simulink model "e05"  (R2023b)
settings: Solver=VariableStepAuto  StartTime=0.0  StopTime=2  RelTol=1e-3
values from neighbouring files (symbols this model uses):
  A = [ ... (first row only)    [e00.m]
  Ad = s1.A    [e00.m]
  B = [ ... (first row only)    [e00.m]
  Bd = s1.B    [e00.m]
  C = [ ... (first row only)    [e00.m]
  Cd = s1.C    [e00.m]
  D = [ ... (first row only)    [e00.m]
  Dd = s1.D    [e00.m]
  Ld = (place(Ad',Cd',p))'    [e00.m]
  Ts = 0.5    [e00.m]
settings Model: Creator=jitbi  LastModifiedBy=Anirvan Krishna

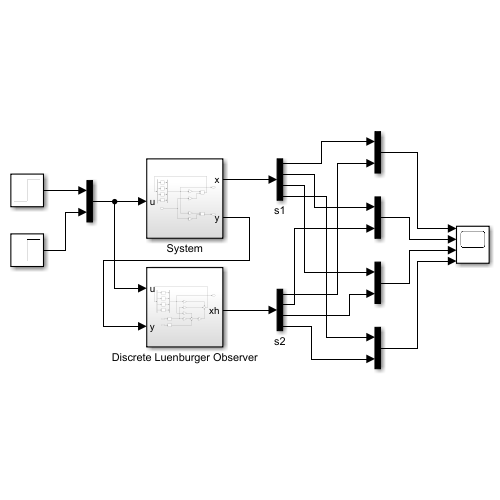
[thumbnail: Simulink's stored preview of the top-level diagram]
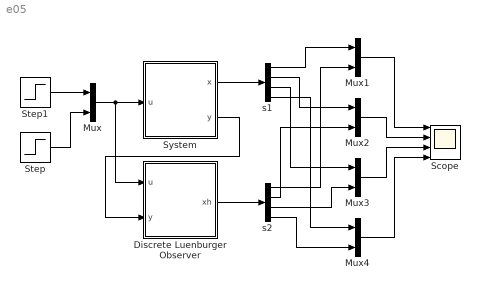
== system e05 ==
  Discrete Luenburger Observer : Subsystem
  Mux{,1..4} (5 alike) : Mux  Inputs=2
  Scope : Scope  NumInputPorts=4
  Step : Step  Time=0  SampleTime=1e-4
  Step1 : Step  Time=0  SampleTime=1e-4
  System : Subsystem
  s1 : Demux
  s2 : Demux
  wires:
  Step/1 -> Mux/2
  Mux/1 -> Discrete Luenburger Observer/1(u), System/1(u)
  Step1/1 -> Mux/1
  System/2(y) -> Discrete Luenburger Observer/2(y)
  System/1(x) -> s1/1
  Discrete Luenburger Observer/1(xh) -> s2/1
  s1/1 -> Mux1/1
  s2/1 -> Mux1/2
  s1/2 -> Mux2/1
  s1/3 -> Mux3/1
  s2/2 -> Mux2/2
  s2/3 -> Mux3/2
  s2/4 -> Mux4/2
  Mux1/1 -> Scope/1
  Mux2/1 -> Scope/2
  Mux3/1 -> Scope/3
  Mux4/1 -> Scope/4
  s1/4 -> Mux4/1

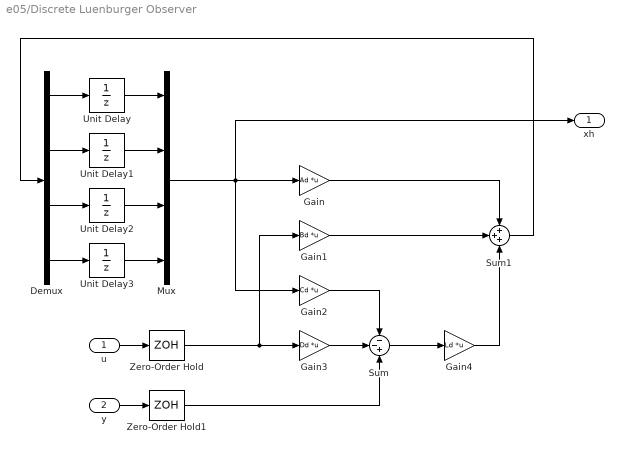
== system e05/Discrete Luenburger Observer ==
  u : Inport
  y : Inport  Port=2
  Demux : Demux
  Gain : Gain  Gain=Ad  Multiplication=Matrix(K*u)
  Gain1 : Gain  Gain=Bd  Multiplication=Matrix(K*u)
  Gain2 : Gain  Gain=Cd  Multiplication=Matrix(K*u)
  Gain3 : Gain  Gain=Dd  Multiplication=Matrix(K*u)
  Gain4 : Gain  Gain=Ld  Multiplication=Matrix(K*u)
  Mux : Mux
  Sum : Sum  Inputs=--+
  Sum1 : Sum  Inputs=+++
  Unit Delay{,1..3} (4 alike) : UnitDelay  SampleTime=Ts  HasFrameUpgradeWarning=on
  Zero-Order Hold : ZeroOrderHold  SampleTime=Ts
  Zero-Order Hold1 : ZeroOrderHold  SampleTime=Ts
  xh : Outport
  wires:
  y/1 -> Zero-Order Hold1/1
  Gain3/1 -> Sum/2
  Unit Delay3/1 -> Mux/4
  Unit Delay1/1 -> Mux/2
  Unit Delay/1 -> Mux/1
  Unit Delay2/1 -> Mux/3
  u/1 -> Zero-Order Hold/1
  Gain4/1 -> Sum1/3
  Demux/2 -> Unit Delay1/1
  Zero-Order Hold/1 -> Gain3/1, Gain1/1
  Mux/1 -> xh/1, Gain2/1, Gain/1
  Demux/4 -> Unit Delay3/1
  Demux/3 -> Unit Delay2/1
  Gain/1 -> Sum1/1
  Demux/1 -> Unit Delay/1
  Zero-Order Hold1/1 -> Sum/3
  Gain1/1 -> Sum1/2
  Sum/1 -> Gain4/1
  Gain2/1 -> Sum/1
  Sum1/1 -> Demux/1

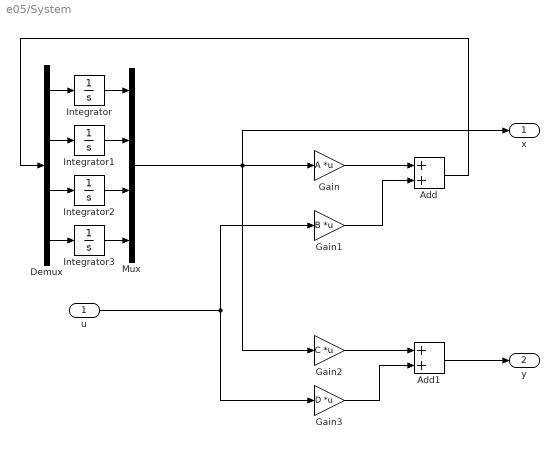
== system e05/System ==
  u : Inport
  Add : Sum
  Add1 : Sum
  Demux : Demux
  Gain : Gain  Gain=A  Multiplication=Matrix(K*u)
  Gain1 : Gain  Gain=B  Multiplication=Matrix(K*u)
  Gain2 : Gain  Gain=C  Multiplication=Matrix(K*u)
  Gain3 : Gain  Gain=D  Multiplication=Matrix(K*u)
  Integrator{,1..3} (4 alike) : Integrator
  Mux : Mux
  x : Outport
  y : Outport  Port=2
  wires:
  Demux/1 -> Integrator/1
  Gain3/1 -> Add1/2
  Integrator/1 -> Mux/1
  u/1 -> Gain3/1, Gain1/1
  Add/1 -> Demux/1
  Demux/3 -> Integrator2/1
  Integrator2/1 -> Mux/3
  Mux/1 -> x/1, Gain/1, Gain2/1
  Demux/4 -> Integrator3/1
  Demux/2 -> Integrator1/1
  Integrator3/1 -> Mux/4
  Integrator1/1 -> Mux/2
  Gain2/1 -> Add1/1
  Gain/1 -> Add/1
  Gain1/1 -> Add/2
  Add1/1 -> y/1
